simulink model "failureInputReadDsrv"  (R2026a)
settings: Solver=ode4  FixedStep=stepSize_s
settings Model: Creator=Edison Altamirano  LastModifiedBy=Edison Altamirano

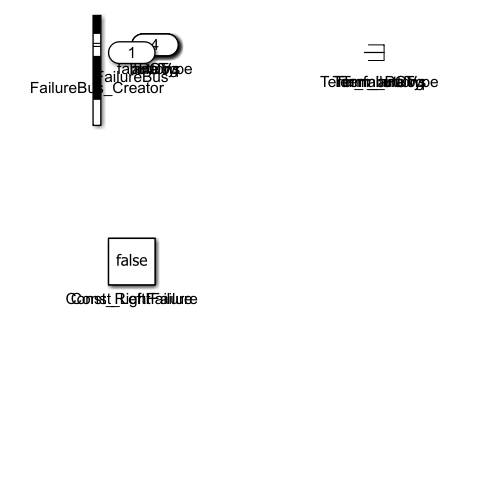
[thumbnail: Simulink's stored preview of the top-level diagram]
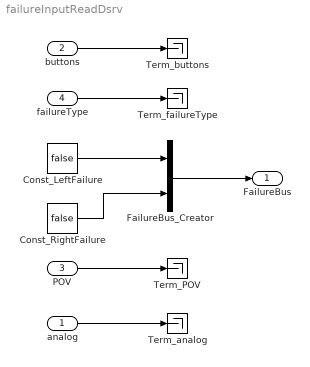
== system failureInputReadDsrv ==
  analog : Inport  PortDimensions=6
  buttons : Inport  Port=2  OutDataTypeStr=uint32
  POV : Inport  Port=3
  failureType : Inport  Port=4  OutDataTypeStr=Enum: EnumHexFailureType
  Const_LeftFailure : Constant  Value=false  OutDataTypeStr=boolean
  Const_RightFailure : Constant  Value=false  OutDataTypeStr=boolean
  FailureBus_Creator : BusCreator  Inputs=2  OutDataTypeStr=Bus: FailureBus
  Term_POV : Terminator
  Term_analog : Terminator
  Term_buttons : Terminator
  Term_failureType : Terminator
  FailureBus : Outport  OutDataTypeStr=Bus: FailureBus
  wires:
  buttons/1 -> Term_buttons/1
  Const_RightFailure/1 -> FailureBus_Creator/2
  Const_LeftFailure/1 -> FailureBus_Creator/1
  failureType/1 -> Term_failureType/1
  FailureBus_Creator/1 -> FailureBus/1
  POV/1 -> Term_POV/1
  analog/1 -> Term_analog/1
